simulink model "pmsm_dynamic_simscape"  (R2016a)
settings: Solver=ode45  StartTime=0.0  StopTime=2  MaxStep=1e-6  RelTol=1e-6
values from neighbouring files (symbols this model uses):
  Kp = Gciabs/abs(1+wz/(2*pi*1000))    [parameters.m]
  L = 0.5e-3    (= 0.0005)    [parameters.m]
  lambda_m = 0.125    [parameters.m]
  P = 8    [parameters.m]
  r = 0.08    [parameters.m]
  Tmref = 240    [parameters.m]
  Vdc = 500    [parameters.m]
  wr = 100*pi*(2/P)    (= 78.5398163397)    [parameters.m]
  wz = wp    (= 160)    [parameters.m]
libraries: powerlib x13, simulink x5
settings Model: Creator=Gorkem  LastModifiedBy=Gorkem
settings GRTTargetCC: GeneratePreprocessorConditionals=Use local settings

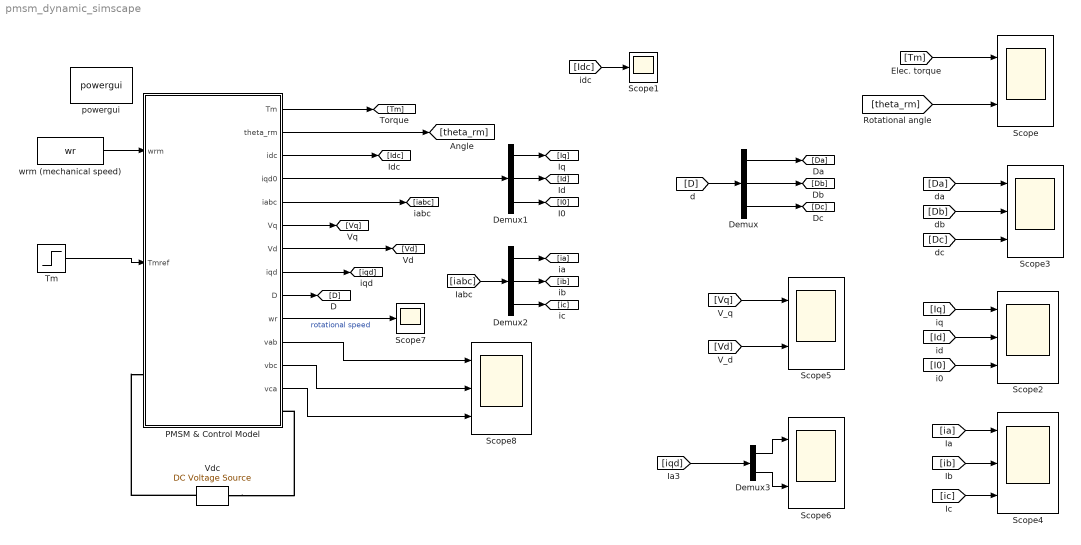
== system pmsm_dynamic_simscape ==
  Demux : Demux  Outputs=3
  Demux1 : Demux  Outputs=3
  Demux2 : Demux  Outputs=3
  Demux3 : Demux  Outputs=2
  PMSM & Control Model : Subsystem
  Scope : Scope  NumInputPorts=2
  Scope1 : Scope
  Scope{2..4,8} (4 alike) : Scope  NumInputPorts=3
  Scope5 : Scope  NumInputPorts=2
  Scope6 : Scope  NumInputPorts=2
  Scope7 : Scope
  Tm : Step  Time=0.4  After=Tmref  SampleTime=0
  Vdc : powerlib/Electrical Sources/DC Voltage Source  Amplitude=Vdc  Measurements=None
  powergui : powerlib/powergui  Priority=1  SimulationMode=Discrete  SolverType=Tustin/Backward Euler (TBE)  SampleTime=1e-6  frequency=60  SPID=off  DisableSnubberDevices=off  DisableRonSwitches=off  DisableVfSwitches=off  SwTol=0  DisplayEquations=off  Interpol=off  ExternalGateDelay=off  methode=off  Ts=10  FunctionMessages=off  echomessages=off  HookPort=off  EnableUseOfTLC=off  x0status=blocks  frequencyindice=0  Pbase=100e6  ErrMax=1e-4  Iterations=50  UnitsV=kV  UnitsW=MW  buscounter=0  RestoreLinks=warning  ResistiveCurrentMeasurement=off  Frange=[0:2:500]  Ylog=off  Xlog=on  ShowGrid=off  save=off  variable=ZData  structure=0  ZoomFFT=off  StartTime=0.0  cycles=1  DisplayStyle=1  fundamental=60  FreqAxis=off  MaxFrequency=1000  frequencyindicesteady=1  RmsSteady=1  display=off
  wrm (mechanical speed) : Constant  Value=wr
  wires:
  wrm (mechanical speed)/1 -> PMSM & Control Model/1(wrm)
  Tm/1 -> PMSM & Control Model/2(Tmref)
  PMSM & Control Model/4(iqd0) -> Demux1/1
  PMSM & Control Model/2(theta_rm) -> [theta_rm]
  PMSM & Control Model/1(Tm) -> [Tm]
  Demux/3 -> [Dc]
  Demux/2 -> [Db]
  Demux/1 -> [Da]
  Demux1/1 -> [Iq]
  Demux1/2 -> [Id]
  Demux1/3 -> [I0]
  PMSM & Control Model/6(Vq) -> [Vq]
  PMSM & Control Model/7(Vd) -> [Vd]
  Demux2/2 -> [ib]
  Demux2/1 -> [ia]
  Demux2/3 -> [ic]
  PMSM & Control Model/3(idc) -> [Idc]
  [Tm] -> Scope/1
  [theta_rm] -> Scope/2
  [Da] -> Scope3/1
  [Db] -> Scope3/2
  [Dc] -> Scope3/3
  [Iq] -> Scope2/1
  [Id] -> Scope2/2
  [I0] -> Scope2/3
  [Idc] -> Scope1/1
  [ia] -> Scope4/1
  [ib] -> Scope4/2
  [ic] -> Scope4/3
  [Vq] -> Scope5/1
  [Vd] -> Scope5/2
  Demux3/1 -> Scope6/1
  Demux3/2 -> Scope6/2
  PMSM & Control Model/10(wr) -> Scope7/1  "rotational speed"
  PMSM & Control Model/5(iabc) -> [iabc]
  [iabc] -> Demux2/1
  PMSM & Control Model/9(D) -> [D]
  [D] -> Demux/1
  PMSM & Control Model/8(iqd) -> [iqd]
  [iqd] -> Demux3/1
  PMSM & Control Model/11(vab) -> Scope8/1
  PMSM & Control Model/12(vbc) -> Scope8/2
  PMSM & Control Model/13(vca) -> Scope8/3
  connections:
  Vdc/RConn1 -- PMSM & Control Model/LConn1
  Vdc/LConn1 -- PMSM & Control Model/RConn1

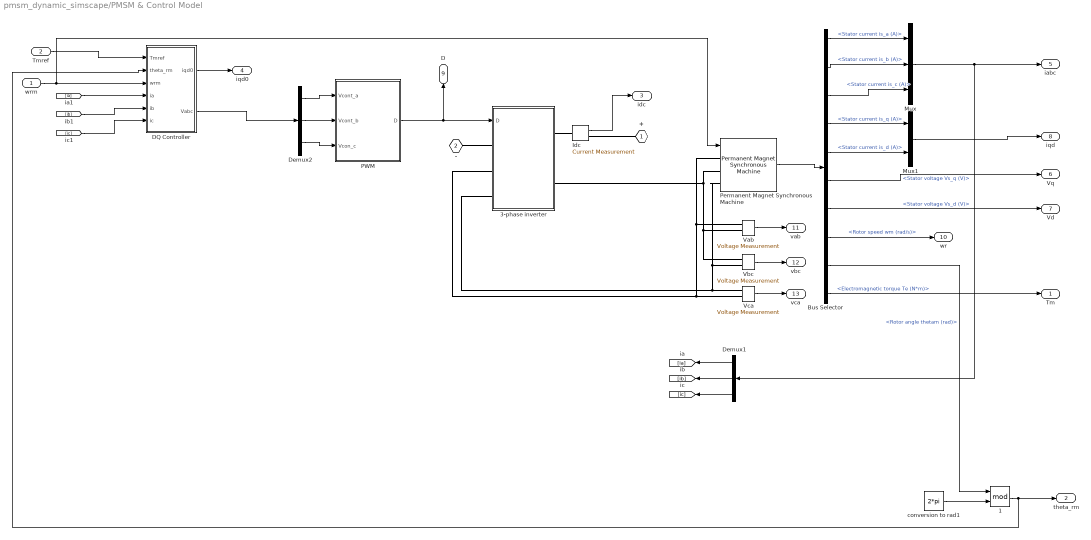
== system pmsm_dynamic_simscape/PMSM & Control Model ==
  wrm : Inport
  Tmref : Inport  Port=2
  "  1" : Math  Operator=mod  SaturateOnIntegerOverflow=on
  3-phase inverter : Subsystem
  Bus Selector : BusSelector  OutputSignals=Stator current is_a (A),Stator current is_b (A),Stator current is_c (A),Stator current is_q (A),Stator current is_d (A),Stator voltage Vs_q (V),Stator voltage Vs_d (V),Rotor speed wm (rad/s),Rotor angle thetam (rad),Electromagnetic torque Te (N*m)
  DQ Controller : Subsystem
  Demux1 : Demux  Outputs=3
  Demux2 : Demux  Outputs=3
  Idc : powerlib/Measurements/Current Measurement  PhasorSimulation=off  OutputType=Complex  PSBequivalent=0
  Mux : Mux  Inputs=3
  Mux1 : Mux  Inputs=2
  PWM : Subsystem
  Permanent Magnet Synchronous Machine : powerlib/Machines/Permanent Magnet Synchronous Machine  NbPhases=3  FluxDistribution=Sinusoidal  RotorType=Salient-pole  MechanicalLoad=Speed w  PresetModel=No  ShowDetailedParameters=on  MeasurementBus=off  Resistance=r  Inductance=8.5e-3  dqInductances=[L,L]  La=0.000395  MachineConstant=Flux linkage established by magnets (V.s)  Flux=lambda_m  VoltageCst=22.6725  TorqueCst=0.1875  Flat=120  Mechanical=[0.0027 0.0004924 P/2 0]  PolePairs=P/2  InitialConditions=[0,0, 0,0]  InitialConditions5ph=[0 0 0 0 0 0]  TsPowergui=0  TsBlock=-1  RefAngle=90 degrees behind phase A axis (modified Park)
  Vab : powerlib/Measurements/Voltage Measurement  PhasorSimulation=off  OutputType=Complex  PSBequivalent=0
  Vbc : powerlib/Measurements/Voltage Measurement  PhasorSimulation=off  OutputType=Complex  PSBequivalent=0
  Vca : powerlib/Measurements/Voltage Measurement  PhasorSimulation=off  OutputType=Complex  PSBequivalent=0
  conversion to rad1 : Constant  Value=2*pi
  + : PMIOPort  Port=1  Side=Left
  - : PMIOPort  Port=2  Side=Right
  Tm : Outport
  theta_rm : Outport  Port=2
  idc : Outport  Port=3
  iqd0 : Outport  Port=4
  iabc : Outport  Port=5
  Vq : Outport  Port=6
  Vd : Outport  Port=7
  iqd : Outport  Port=8
  D : Outport  Port=9
  wr : Outport  Port=10
  vab : Outport  Port=11
  vbc : Outport  Port=12
  vca : Outport  Port=13
  wires:
  DQ Controller/2(Vabc) -> Demux2/1
  Idc/1 -> idc/1
  wrm/1 -> Permanent Magnet Synchronous Machine/1, DQ Controller/3(wrm)
  DQ Controller/1(iqd0) -> iqd0/1
  Demux1/1 -> [ia]
  Demux1/2 -> [ib]
  Demux1/3 -> [ic]
  Demux2/1 -> PWM/1(Vcont_a)
  Demux2/2 -> PWM/2(Vcont_b)
  Demux2/3 -> PWM/3(Vcon_c)
  Permanent Magnet Synchronous Machine/1 -> Bus Selector/1
  Bus Selector/1 -> Mux/1  "<Stator current is_a (A)>"
  Bus Selector/2 -> Mux/2  "<Stator current is_b (A)>"
  Bus Selector/3 -> Mux/3  "<Stator current is_c (A)>"
  Mux/1 -> Demux1/1, iabc/1
  Bus Selector/4 -> Mux1/1  "<Stator current is_q (A)>"
  Bus Selector/5 -> Mux1/2  "<Stator current is_d (A)>"
  Mux1/1 -> iqd/1
  Bus Selector/6 -> Vq/1  "<Stator voltage Vs_q (V)>"
  Bus Selector/7 -> Vd/1  "<Stator voltage Vs_d (V)>"
  Bus Selector/10 -> Tm/1  "<Electromagnetic torque Te (N*m)>"
  Bus Selector/9 -> "  1"/1  "<Rotor angle thetam (rad)>"
  [ia] -> DQ Controller/4(ia)
  [ib] -> DQ Controller/5(ib)
  [ic] -> DQ Controller/6(ic)
  PWM/1(D) -> D/1, 3-phase inverter/1(D)
  Tmref/1 -> DQ Controller/1(Tmref)
  conversion to rad1/1 -> "  1"/2
  "  1"/1 -> theta_rm/1, DQ Controller/2(theta_rm)
  Bus Selector/8 -> wr/1  "<Rotor speed wm (rad/s)>"
  Vab/1 -> vab/1
  Vbc/1 -> vbc/1
  Vca/1 -> vca/1
  connections:
  -/RConn1 -- 3-phase inverter/LConn1
  Idc/LConn1 -- 3-phase inverter/RConn1
  Idc/RConn1 -- +/RConn1
  Permanent Magnet Synchronous Machine/LConn1 -- Vca/LConn2 -- 3-phase inverter/LConn2 -- Vab/LConn1
  Permanent Magnet Synchronous Machine/LConn2 -- Vbc/LConn1 -- Vab/LConn2 -- 3-phase inverter/RConn2
  Permanent Magnet Synchronous Machine/LConn3 -- 3-phase inverter/LConn3 -- Vca/LConn1 -- Vbc/LConn2

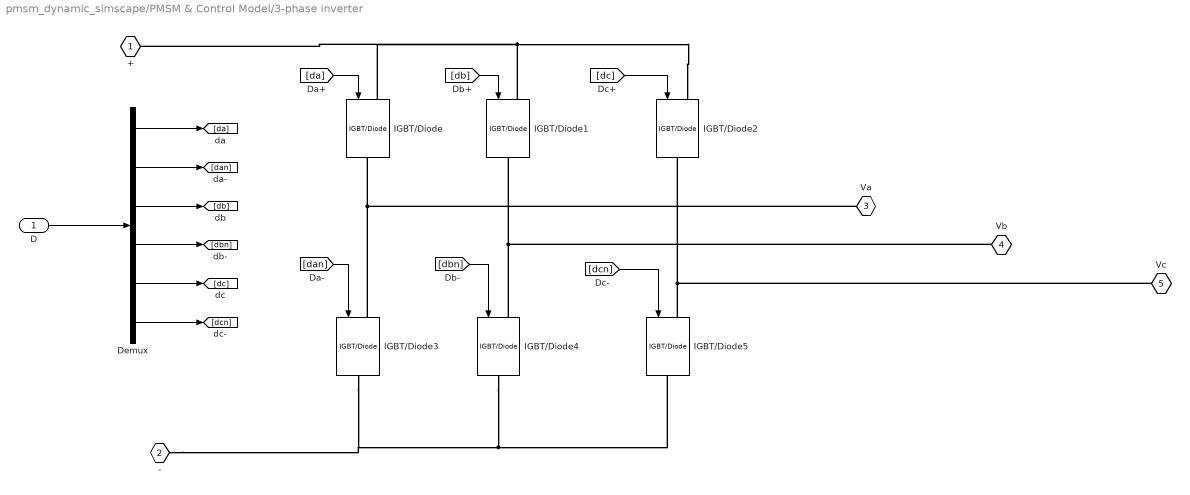
== system pmsm_dynamic_simscape/PMSM & Control Model/3-phase inverter ==
  D : Inport
  Demux : Demux  Outputs=6
  IGBT/Diode{,1..5} (6 alike) : powerlib/Power Electronics/IGBT//Diode  Ron=1e-3  Rs=1e5  Cs=inf  Measurements=off
  + : PMIOPort  Port=1  Side=Right
  - : PMIOPort  Port=2  Side=Left
  Va : PMIOPort  Port=3  Side=Left
  Vb : PMIOPort  Port=4  Side=Right
  Vc : PMIOPort  Port=5  Side=Left
  wires:
  D/1 -> Demux/1
  Demux/1 -> [da]
  Demux/2 -> [dan]
  Demux/3 -> [db]
  Demux/4 -> [dbn]
  Demux/5 -> [dc]
  Demux/6 -> [dcn]
  [da] -> IGBT/Diode/1
  [dan] -> IGBT/Diode3/1
  [dbn] -> IGBT/Diode4/1
  [dcn] -> IGBT/Diode5/1
  [db] -> IGBT/Diode1/1
  [dc] -> IGBT/Diode2/1
  connections:
  IGBT/Diode1/LConn1 -- IGBT/Diode2/LConn1 -- +/RConn1 -- IGBT/Diode/LConn1
  IGBT/Diode4/RConn1 -- IGBT/Diode5/RConn1 -- -/RConn1 -- IGBT/Diode3/RConn1
  IGBT/Diode3/LConn1 -- Va/RConn1 -- IGBT/Diode/RConn1
  IGBT/Diode4/LConn1 -- Vb/RConn1 -- IGBT/Diode1/RConn1
  IGBT/Diode5/LConn1 -- Vc/RConn1 -- IGBT/Diode2/RConn1

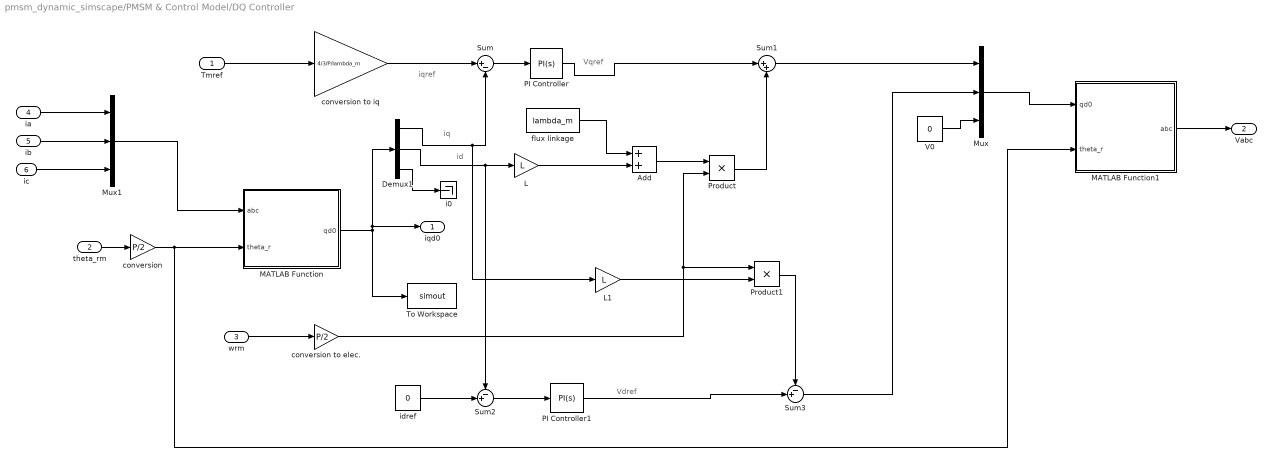
== system pmsm_dynamic_simscape/PMSM & Control Model/DQ Controller ==
  note: iqref
  note: Vdref
  note: id
  note: Vqref
  note: iq
  Tmref : Inport
  theta_rm : Inport  Port=2
  wrm : Inport  Port=3
  ia : Inport  Port=4
  ib : Inport  Port=5
  ic : Inport  Port=6
  Add : Sum
  Demux1 : Demux  Outputs=[1 1 1]
  L : Gain  Gain=L
  L1 : Gain  Gain=L
  MATLAB Function : MATLAB Function  TreatAsAtomicUnit=on
  MATLAB Function1 : MATLAB Function  TreatAsAtomicUnit=on
  Mux : Mux  Inputs=[1 1 1]
  Mux1 : Mux  Inputs=[1 1 1]
  PI Controller : simulink/Continuous/PID Controller  Controller=PI  TimeDomain=Continuous-time  SampleTime=-1  IntegratorMethod=Forward Euler  FilterMethod=Forward Euler  Form=Parallel  UseFilter=on  ControllerParametersSource=internal  P=Kp  I=Kp*wz  D=-5  N=1  InitialConditionSource=internal  InitialConditionForIntegrator=0  InitialConditionForFilter=0  ExternalReset=none  LimitOutput=off  UpperSaturationLimit=inf  LowerSaturationLimit=-inf  LinearizeAsGain=on  AntiWindupMode=none  Kb=1  TrackingMode=off  Kt=1  PParamMin=[]  PParamMax=[]  IParamMin=[]  IParamMax=[]  DParamMin=[]  DParamMax=[]  NParamMin=[]  NParamMax=[]  KbParamMin=[]  KbParamMax=[]  KtParamMin=[]  KtParamMax=[]  POutMin=[]  POutMax=[]  IOutMin=[]  IOutMax=[]  DOutMin=[]  DOutMax=[]  NOutMin=[]  NOutMax=[]  KbOutMin=[]  KbOutMax=[]  KtOutMin=[]  KtOutMax=[]  IntegratorOutMin=[]  IntegratorOutMax=[]  FilterOutMin=[]  FilterOutMax=[]  SumOutMin=[]  SumOutMax=[]  SumI1OutMin=[]  SumI1OutMax=[]  SumI2OutMin=[]  SumI2OutMax=[]  SumI3OutMin=[]  SumI3OutMax=[]  SumDOutMin=[]  SumDOutMax=[]  SaturationOutMin=[]  SaturationOutMax=[]  IntegratorContinuousStateAttributes=''  IntegratorStateMustResolveToSignalObject=off  IntegratorRTWStateStorageClass=Auto  FilterContinuousStateAttributes=''  FilterStateMustResolveToSignalObject=off  FilterRTWStateStorageClass=Auto  DifferentiatorICPrevScaledInput=0  DifferentiatorOutMin=[]  DifferentiatorOutMax=[]
  PI Controller1 : simulink/Continuous/PID Controller  Controller=PI  TimeDomain=Continuous-time  SampleTime=-1  IntegratorMethod=Forward Euler  FilterMethod=Forward Euler  Form=Parallel  UseFilter=on  ControllerParametersSource=internal  P=Kp  I=Kp*wz  D=-5  N=1  InitialConditionSource=internal  InitialConditionForIntegrator=0  InitialConditionForFilter=0  ExternalReset=none  LimitOutput=off  UpperSaturationLimit=inf  LowerSaturationLimit=-inf  LinearizeAsGain=on  AntiWindupMode=none  Kb=1  TrackingMode=off  Kt=1  PParamMin=[]  PParamMax=[]  IParamMin=[]  IParamMax=[]  DParamMin=[]  DParamMax=[]  NParamMin=[]  NParamMax=[]  KbParamMin=[]  KbParamMax=[]  KtParamMin=[]  KtParamMax=[]  POutMin=[]  POutMax=[]  IOutMin=[]  IOutMax=[]  DOutMin=[]  DOutMax=[]  NOutMin=[]  NOutMax=[]  KbOutMin=[]  KbOutMax=[]  KtOutMin=[]  KtOutMax=[]  IntegratorOutMin=[]  IntegratorOutMax=[]  FilterOutMin=[]  FilterOutMax=[]  SumOutMin=[]  SumOutMax=[]  SumI1OutMin=[]  SumI1OutMax=[]  SumI2OutMin=[]  SumI2OutMax=[]  SumI3OutMin=[]  SumI3OutMax=[]  SumDOutMin=[]  SumDOutMax=[]  SaturationOutMin=[]  SaturationOutMax=[]  IntegratorContinuousStateAttributes=''  IntegratorStateMustResolveToSignalObject=off  IntegratorRTWStateStorageClass=Auto  FilterContinuousStateAttributes=''  FilterStateMustResolveToSignalObject=off  FilterRTWStateStorageClass=Auto  DifferentiatorICPrevScaledInput=0  DifferentiatorOutMin=[]  DifferentiatorOutMax=[]
  Product : Product
  Product1 : Product
  Sum : Sum  Inputs=|+-
  Sum1 : Sum  Inputs=|++
  Sum2 : Sum  Inputs=-+|
  Sum3 : Sum  Inputs=-+|
  To Workspace : ToWorkspace  VariableName=simout  SaveFormat=Structure  SampleTime=-1
  V0 : Constant  Value=0
  "conversion " : Gain  Gain=P/2
  conversion to elec. : Gain  Gain=P/2
  conversion to iq : Gain  Gain=4/3/P/lambda_m
  flux linkage : Constant  Value=lambda_m
  i0 : Terminator
  idref : Constant  Value=0
  iqd0 : Outport
  Vabc : Outport  Port=2
  wires:
  wrm/1 -> conversion to elec./1
  theta_rm/1 -> "conversion "/1
  Tmref/1 -> conversion to iq/1
  MATLAB Function/1(qd0) -> Demux1/1, iqd0/1, To Workspace/1
  Demux1/1 -> Sum/2, L1/1
  PI Controller/1 -> Sum1/1
  Demux1/2 -> Sum2/1, L/1
  L/1 -> Add/2
  flux linkage/1 -> Add/1
  Add/1 -> Product/1
  conversion to elec./1 -> Product/2, Product1/1
  idref/1 -> Sum2/2
  Sum2/1 -> PI Controller1/1
  L1/1 -> Product1/2
  PI Controller1/1 -> Sum3/2
  Sum1/1 -> Mux/1
  V0/1 -> Mux/3
  "conversion "/1 -> MATLAB Function1/2(theta_r), MATLAB Function/2(theta_r)
  Demux1/3 -> i0/1
  Mux1/1 -> MATLAB Function/1(abc)
  Sum3/1 -> Mux/2
  Mux/1 -> MATLAB Function1/1(qd0)
  MATLAB Function1/1(abc) -> Vabc/1
  ia/1 -> Mux1/1
  ib/1 -> Mux1/2
  ic/1 -> Mux1/3
  Product/1 -> Sum1/2
  Product1/1 -> Sum3/1
  conversion to iq/1 -> Sum/1
  Sum/1 -> PI Controller/1

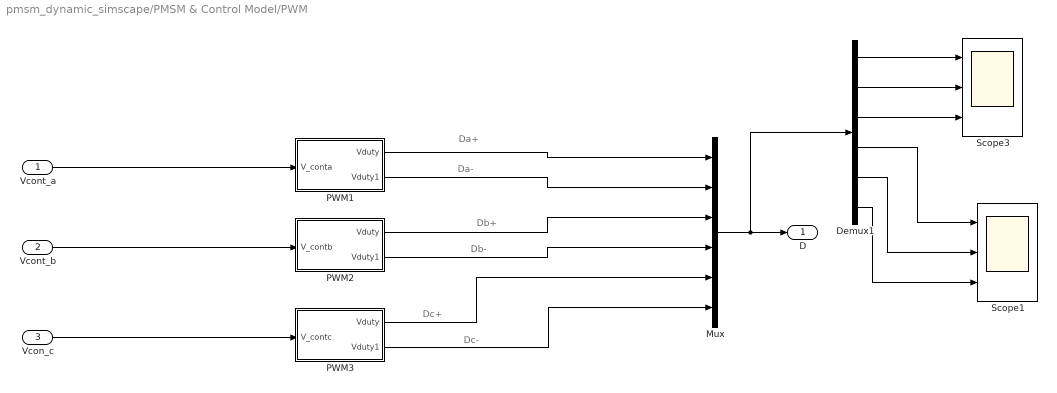
== system pmsm_dynamic_simscape/PMSM & Control Model/PWM ==
  note: Dc-
  note: Dc+
  note: Db-
  note: Db+
  note: Da-
  note: Da+
  Vcont_a : Inport
  Vcont_b : Inport  Port=2
  Vcon_c : Inport  Port=3
  Demux1 : Demux  Outputs=6
  Mux : Mux  Inputs=6
  PWM1 : Subsystem
  PWM2 : Subsystem
  PWM3 : Subsystem
  Scope1 : Scope  NumInputPorts=3
  Scope3 : Scope  NumInputPorts=3
  D : Outport
  wires:
  Mux/1 -> Demux1/1, D/1
  Demux1/1 -> Scope3/1
  Demux1/2 -> Scope3/2
  Demux1/3 -> Scope3/3
  Demux1/4 -> Scope1/1
  Demux1/5 -> Scope1/2
  Demux1/6 -> Scope1/3
  PWM1/2(Vduty1) -> Mux/2
  PWM2/2(Vduty1) -> Mux/4
  PWM3/2(Vduty1) -> Mux/6
  Vcon_c/1 -> PWM3/1(V_contc)
  Vcont_a/1 -> PWM1/1(V_conta)
  PWM1/1(Vduty) -> Mux/1
  Vcont_b/1 -> PWM2/1(V_contb)
  PWM2/1(Vduty) -> Mux/3
  PWM3/1(Vduty) -> Mux/5

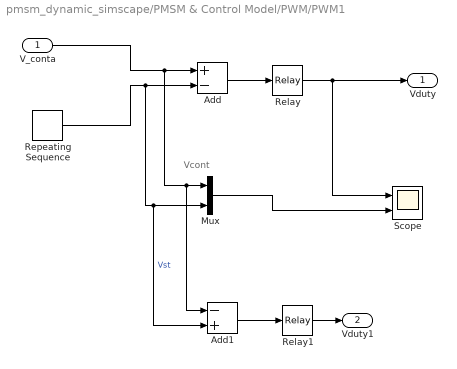
== system pmsm_dynamic_simscape/PMSM & Control Model/PWM/PWM1 ==
  note: Vcont
  V_conta : Inport
  Add : Sum  Inputs=+-
  Add1 : Sum  Inputs=-+
  Mux : Mux  Inputs=2
  Relay : Relay  ZeroCross=off
  Relay1 : Relay  ZeroCross=off
  Repeating Sequence : simulink/Sources/Repeating Sequence  rep_seq_t=[0 0.5e-5 1e-5]  rep_seq_y=[50 0 50]
  Scope : Scope  NumInputPorts=2
  Vduty : Outport
  Vduty1 : Outport  Port=2
  wires:
  Relay/1 -> Vduty/1, Scope/1
  Repeating Sequence/1 -> Add1/2, Mux/2, Add/2  "Vst"
  Add/1 -> Relay/1
  Mux/1 -> Scope/2
  V_conta/1 -> Add1/1, Mux/1, Add/1
  Add1/1 -> Relay1/1
  Relay1/1 -> Vduty1/1

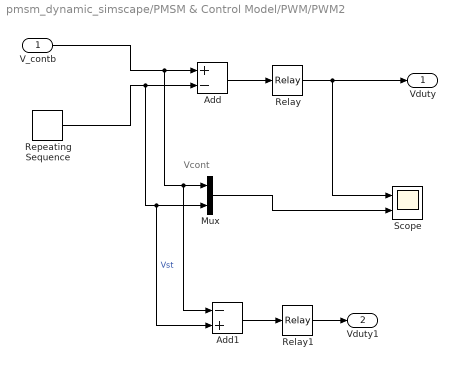
== system pmsm_dynamic_simscape/PMSM & Control Model/PWM/PWM2 ==
  note: Vcont
  V_contb : Inport
  Add : Sum  Inputs=+-
  Add1 : Sum  Inputs=-+
  Mux : Mux  Inputs=2
  Relay : Relay  ZeroCross=off
  Relay1 : Relay  ZeroCross=off
  Repeating Sequence : simulink/Sources/Repeating Sequence  rep_seq_t=[0 0.5e-5 1e-5]  rep_seq_y=[50 0 50]
  Scope : Scope  NumInputPorts=2
  Vduty : Outport
  Vduty1 : Outport  Port=2
  wires:
  Relay/1 -> Vduty/1, Scope/1
  Repeating Sequence/1 -> Add1/2, Mux/2, Add/2  "Vst"
  Add/1 -> Relay/1
  Mux/1 -> Scope/2
  V_contb/1 -> Add1/1, Mux/1, Add/1
  Add1/1 -> Relay1/1
  Relay1/1 -> Vduty1/1

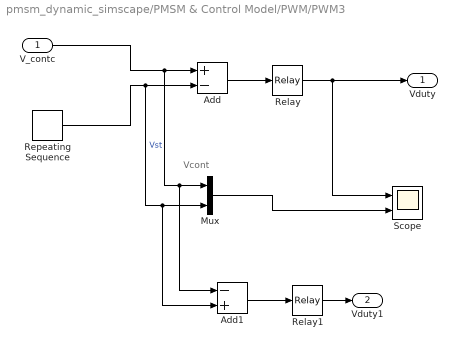
== system pmsm_dynamic_simscape/PMSM & Control Model/PWM/PWM3 ==
  note: Vcont
  V_contc : Inport
  Add : Sum  Inputs=+-
  Add1 : Sum  Inputs=-+
  Mux : Mux  Inputs=2
  Relay : Relay  ZeroCross=off
  Relay1 : Relay  ZeroCross=off
  Repeating Sequence : simulink/Sources/Repeating Sequence  rep_seq_t=[0 0.5e-5 1e-5]  rep_seq_y=[50 0 50]
  Scope : Scope  NumInputPorts=2
  Vduty : Outport
  Vduty1 : Outport  Port=2
  wires:
  Relay/1 -> Vduty/1, Scope/1
  Repeating Sequence/1 -> Add1/2, Mux/2, Add/2  "Vst"
  Add/1 -> Relay/1
  Mux/1 -> Scope/2
  V_contc/1 -> Add1/1, Mux/1, Add/1
  Add1/1 -> Relay1/1
  Relay1/1 -> Vduty1/1

== matlab function pmsm_dynamic_simscape/PMSM & Control Model/DQ Controller/MATLAB Function1 ==
  data: qd0 input; abc output; theta_r input
function abc = Inverse_DQTransform(qd0, theta_r)
%#codegen

Kr = 2/3*[  cos(theta_r)      cos(theta_r-2*pi/3)     cos(theta_r + 2*pi/3);
            sin(theta_r)      sin(theta_r-2*pi/3)     sin(theta_r + 2*pi/3);
            1/2               1/2                     1/2];
  
abc = Kr\qd0;

== matlab function pmsm_dynamic_simscape/PMSM & Control Model/DQ Controller/MATLAB Function ==
  data: abc input; qd0 output; theta_r input
function qd0 = DQTransform(abc, theta_r)
%#codegen

Kr = 2/3*[  cos(theta_r)      cos(theta_r-2*pi/3)     cos(theta_r + 2*pi/3);
            sin(theta_r)      sin(theta_r-2*pi/3)     sin(theta_r + 2*pi/3);
            1/2               1/2                     1/2];
  
qd0 = Kr*abc;
